simulink model "GEMM_Ex2"  (R2025a)
settings: Solver=VariableStepAuto  StartTime=0.0  StopTime=10  RelTol=1e-3
undefined symbols (not defined in the file): Correlation_ValidMode, DUT, L, major, Row, vsva1596, xcvc1702
libraries: aieUtilities x2, aieDSP x1, vmcUtilities x1
settings Model: Creator=sdegala  LastModifiedBy=robg
settings ModelReferenceCC: EnableRefExpFcnMdlSchedulingChecks=on
settings RTWCC: GPUComputeCapability=3.5

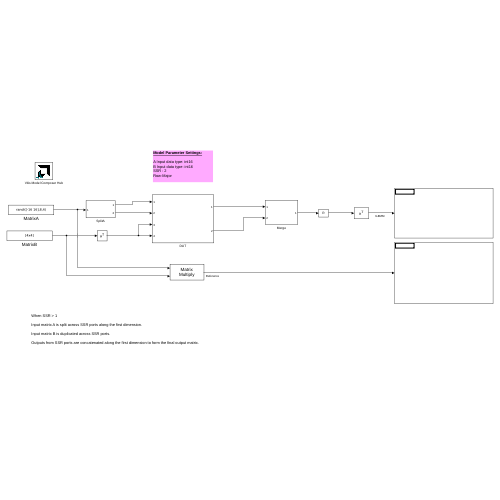
[thumbnail: Simulink's stored preview of the top-level diagram]
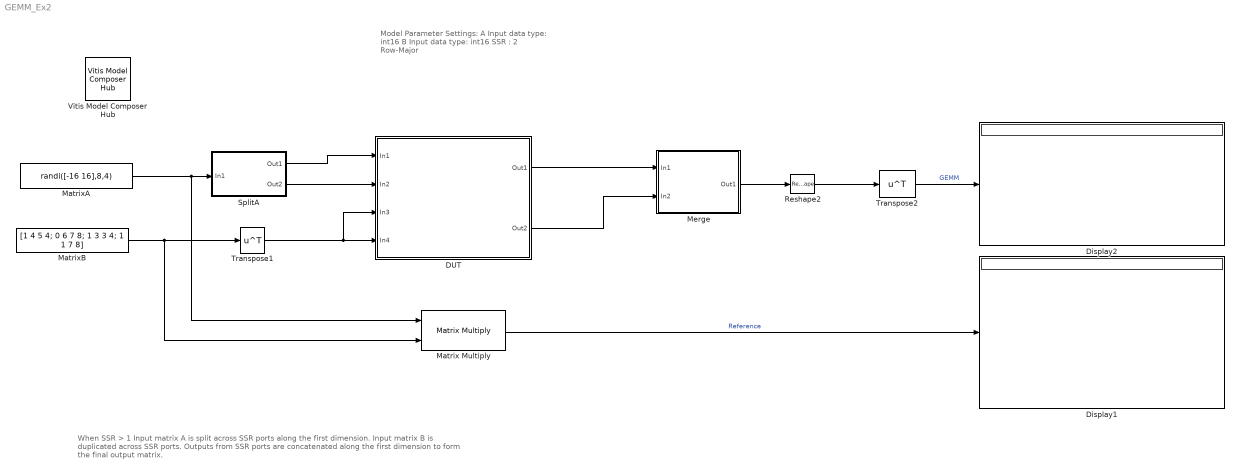
== system GEMM_Ex2 ==
  note: When SSR > 1
      |
      | Input matrix A is split across SSR ports along the first dimension.
      |
      | Input matrix B is duplicated across SSR ports.
      |
      | Outputs from SSR ports are concatenated along the first dimension to form the final output matrix.
  note: Model Parameter Settings:
      |
      | A Input data type: int16
      | B Input data type: int16
      | SSR : 2
      | Row-Major
  DUT : Subsystem
  Display1 : Display
  Display2 : Display
  Matrix Multiply : Product  Multiplication=Matrix(*)  OutDataTypeStr=int16
  MatrixA : Constant  Value=randi([-16 16],8,4)  OutDataTypeStr=int16  SampleTime=1
  MatrixB : Constant  Value=[1 4 5 4; 0 6 7 8; 1 3 3 4; 1 1 7 8]  OutDataTypeStr=int16  SampleTime=1
  Merge : Subsystem
  Reshape2 : Reshape  OutputDimensionality=Customize  OutputDimensions=[4,8]
  SplitA : Subsystem
  Transpose1 : Math  Operator=transpose
  Transpose2 : Math  Operator=transpose
  Vitis Model Composer Hub : vmcUtilities/Vitis Model Composer Hub  Tag=genX  CodeGeneration=off  SubsystemName=DUT  BlockHierPath=Correlation_ValidMode/DUT  SubsystemType=AIENode  StartColumn=1  NumberOfColumns=1  TargetDirectory=./code  exportDesign=off  analyzeDesign=on  validateDesignOnHw=off  ExportType=AI Engines  IpVendor=xilinx.com  IpLibrary=hls  IpVersion=1.0  IpHWLanguage=Verilog  AieCompilerOptions={}  AieSimulatorOptions={}  AieGraphIterations=-1  CreateTestbench=on  TestbenchStackSize=10  RunRtlSim=off  RunCSim=off  RunAieSim=off  AieSimTimeout=50000  RunAieSimProfiling=off  LaunchVitisAnalyzer=off  PlotOutput=off  RunX86Sim=off  X86SimTimeout=10  GenHwImage=off  GenLibadfXo=off  GenHwValidationCode=off  PlatformType=Not Specified  HwSystemType=Baremetal  HwValidationTarget=hw  ProjDevice=xcvc1702-vsva1596-2LP-e-L  ProjDevicePart=xcvc1702-vsva1596-2LP-e-L  AIEType=AIE  SamplePeriod=-1  ClockFrequency=200  DataPathParallelism=1  xilinxfamily=versalaicore  part=xcvc1702  speed=-2LP-e-L  package=vsva1596  directory=./netlist  testbench=off  incr_netlist=off  synthesis_tool=Vivado  clock_wrapper=Clock Enables  dbl_ovrd=According to Block Masks  dcm_input_clock_period=10  sysclk_period=10  simulink_period=1  eval_field=0  IPInfoJsonString="{\"DUTSubsystemName\":\"DUT\",\"AIESubsystem\":{\"SubsystemName\":\"DUT\",\"TargetDirectory\":\"./code\",\"AIEArrayConfig\":\"Use entire AIE array\",\"StartColumn\":\"0\",\"NumberOfColumns\":\"1\"},\"SubsystemTag\":\"AIENode\"}"  LogFileName=/proj/xhdhdstaff5/sdegala/Head1/HEAD/2025_2_work/AIE_BLOCKS_2025_2/code/model_composer.log  NThreads=4  IPConfigFile=/tmp/vmctmp-11198269997411262707/Correlation_ValidMode_ipconfig.json
  wires:
  MatrixB/1 -> Matrix Multiply/2, Transpose1/1
  MatrixA/1 -> Matrix Multiply/1, SplitA/1(In1)
  Matrix Multiply/1 -> Display1/1  "Reference"
  Transpose2/1 -> Display2/1  "GEMM"
  Reshape2/1 -> Transpose2/1
  Merge/1(Out1) -> Reshape2/1
  SplitA/1(Out1) -> DUT/1(In1)
  SplitA/2(Out2) -> DUT/2(In2)
  Transpose1/1 -> DUT/3(In3), DUT/4(In4)
  DUT/1(Out1) -> Merge/1(In1)
  DUT/2(Out2) -> Merge/2(In2)

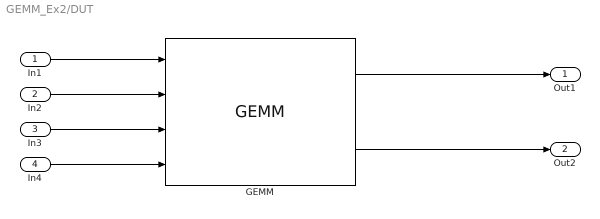
== system GEMM_Ex2/DUT ==
  In1 : Inport
  In2 : Inport  Port=2
  In3 : Inport  Port=3
  In4 : Inport  Port=4
  GEMM : aieDSP/GEMM  AIE_VARIANT=1  data_type_A=int16  data_type_B=int16  data_type_out=int16  Dim_A=8  Dim_B=4  Dim_AB=4  ssr=2  casc_length=1  InputWindowSizeA=32  InputWindowSizeB=16  A_Leading_data=Row-major(0)  B_Leading_data=Row-major(0)  Output_Leading_data=Row-major(0)  A_Tiling_data=off  B_Tiling_data=off  Output_Detiling_data=off  shift_output=0  rnd_mode=Floor  sat_mode=None  blockJsonConstraints=[]  blockJsonConstraintsInternal=[]  spec=vmc_matrix_mult.json  SerializedMaskParamNames=[]  SerializedMaskParamValues=[]  SerializedMaskParamVisibilities=[]  block_type=GEMM  SerializedMaskParamDataypes=uint|typename|typename|typename|uint|uint|uint|uint|uint|uint|uint|uint|uint|uint|uint|uint|uint|uint|uint|uint  SerializedMaskParamEnumStrArr=0|0|0|0|0|0|0|0|0|0|0|Row-major(0),Column-major(1)|Row-major(0),Column-major(1)|Row-major(0),Column-major(1)|0|0|0|0|Floor,Ceiling,Round to positive infinity,Round to negative infinity,Round symmetrical to infinity,Round symmetrical to zero,Round convergent to even,Round convergent to odd|None,Saturate,Symmetric  SerializedMaskParamEnumValArr=0|0|0|0|0|0|0|0|0|0|0|0,1|0,1|0,1|0|0|0|0|0,1,2,3,4,5,6,7|0,1,3  SerializedMaskParamVectorArr=0|0|0|0|0|0|0|0|0|0|0|0|0|0|0|0|0|0|0|0  SerializedMaskParamKeys=AIE_VARIANT|TT_DATA_A|TT_DATA_B|TT_OUT_DATA|TP_DIM_A|TP_DIM_B|TP_DIM_AB|TP_SSR|TP_CASC_LEN|TP_INPUT_WINDOW_VSIZE_A|TP_INPUT_WINDOW_VSIZE_B|TP_DIM_A_LEADING|TP_DIM_B_LEADING|TP_DIM_OUT_LEADING|TP_ADD_TILING_A|TP_ADD_TILING_B|TP_ADD_DETILING_OUT|TP_SHIFT|TP_RND|TP_SAT
  Out1 : Outport
  Out2 : Outport  Port=2
  wires:
  In3/1 -> GEMM/3
  GEMM/2 -> Out2/1
  In1/1 -> GEMM/1
  GEMM/1 -> Out1/1
  In2/1 -> GEMM/2
  In4/1 -> GEMM/4

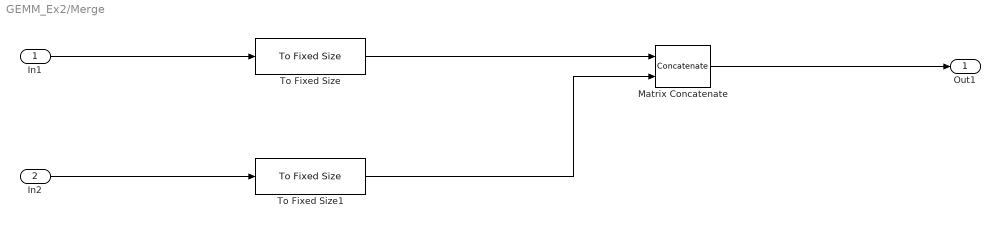
== system GEMM_Ex2/Merge ==
  In1 : Inport
  In2 : Inport  Port=2
  Matrix Concatenate : Concatenate  Mode=Multidimensional array
  To Fixed Size : aieUtilities/To Fixed Size  Mode=Stop simulation when input variable-size signal is not full  OutputSize=Inherit: Same as input  CopyMethod=Buffer samples to form output  HasStatusOutput=on
  To Fixed Size1 : aieUtilities/To Fixed Size  Mode=Stop simulation when input variable-size signal is not full  OutputSize=Inherit: Same as input  CopyMethod=Buffer samples to form output  HasStatusOutput=on
  Out1 : Outport
  wires:
  In1/1 -> To Fixed Size/1
  In2/1 -> To Fixed Size1/1
  Matrix Concatenate/1 -> Out1/1
  To Fixed Size/1 -> Matrix Concatenate/1
  To Fixed Size1/1 -> Matrix Concatenate/2

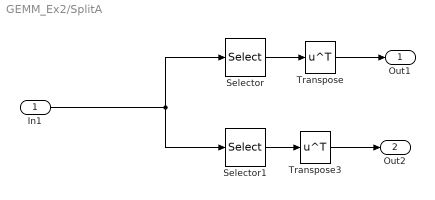
== system GEMM_Ex2/SplitA ==
  In1 : Inport
  Selector : Selector  NumberOfDimensions=2  InputPortWidth=3  IndexOptions=Index vector (dialog),Index vector (dialog)  Indices=1:4,1:4  OutputSizes=1,1
  Selector1 : Selector  NumberOfDimensions=2  InputPortWidth=3  IndexOptions=Index vector (dialog),Index vector (dialog)  Indices=5:8,1:4  OutputSizes=1,1
  Transpose : Math  Operator=transpose
  Transpose3 : Math  Operator=transpose
  Out1 : Outport
  Out2 : Outport  Port=2
  wires:
  Selector1/1 -> Transpose3/1
  Selector/1 -> Transpose/1
  Transpose3/1 -> Out2/1
  Transpose/1 -> Out1/1
  In1/1 -> Selector/1, Selector1/1
